simulink model "s_tanks_2_edit"  (R2021a)
settings: Solver=ode4  StartTime=0.0  StopTime=60  FixedStep=0.002  RelTol=1e-3  EnableMultiTasking=on
undefined symbols (not defined in the file or in its folder): Ao1, Ao2, At1, At2, g, Kff_2, Ki_1, Ki_2, Kp, Kp_1, Kp_2, L20, LR_1_MAX, MAX_L1_WDUP, MAX_L2_WDUP, TS, VMAX_AMP
settings Model: ExtModeTrigDuration=60000  Creator=MLevis  LastModifiedBy=tronc
settings SolverCC: AlgebraicLoopSolver=TrustRegion  PositivePriorityOrder=on
settings DataIOCC: LimitDataPoints=on  SaveFormat=Array  SignalLoggingSaveFormat=ModelDataLogs  ReturnWorkspaceOutputs=off
settings OptimizationCC: ExpressionDepthLimit=2147483647  InitFltsAndDblsToZero=on  LifeSpan=inf
settings DebuggingCC: SaveWithParameterizedLinksMsg=none  UnderspecifiedInitializationDetection=Classic  MergeDetectMultiDrivingBlocksExec=none  SolverPrmCheckMsg=warning  FcnCallInpInsideContextMsg=warning  StateNameClashWarn=warning  SFUnexpectedBacktrackingDiag=warning  SFNoUnconditionalDefaultTransitionDiag=warning  SFExecutionAtInitializationDiag=none  SFMachineParentedDataDiag=warning  ArithmeticOperatorsInVariantConditions=warning
settings HardwareCC: ProdBitPerPointer=32  ProdBitPerSizeT=32  ProdBitPerPtrDiffT=32  ProdLargestAtomicFloat=None  ProdIntDivRoundTo=Undefined  ProdEndianess=Unspecified  ProdWordSize=32  ProdHWDeviceType=32-bit Generic
settings ModelReferenceCC: PropagateSignalLabelsOutOfModel=off
settings SFSimCC: SimUseLocalCustomCode=off  CustomCodeUndefinedFunction=UseInterfaceOnly
settings RTWCC: Description=QuaRC Win32 Target  SystemTargetFile=quarc_windows.tlc  TemplateMakefile=quarc_default_tmf  RTWUseLocalCustomCode=off
settings CodeAppCC: StateflowObjectComments=on
settings STFCustomTargetCC: TargetFcnLib=ansi_tfl_tmw.mat  TargetPreCompLibLocation=C:\PROGRA~3\QUARC\lib\2012b\windows\release  CPPClassGenCompliant=on  UseToolchainInfoCompliant=off  SystemTargetFile=quarc_windows.tlc
settings GRTTargetCC: TargetFcnLib=ansi_tfl_tmw.mat  TargetPreCompLibLocation=C:\PROGRA~3\QUARC\lib\2012b\windows\release  TargetLangStandard=C89/C90 (ANSI)  ParMdlRefBuildCompliant=off  CompOptLevelCompliant=off  ConcurrentExecutionCompliant=off  CombineOutputUpdateFcns=off  MatFileLogging=off  GRTInterface=on  UseToolchainInfoCompliant=off  ExtMode=on  ExtModeMexFile=quarc_comm
settings ConfigComp: CovMetricSettings=dw  CovSaveCumulativeToWorkspaceVar=on  CovSaveSingleToWorkspaceVar=on  CovExternalEMLEnable=off

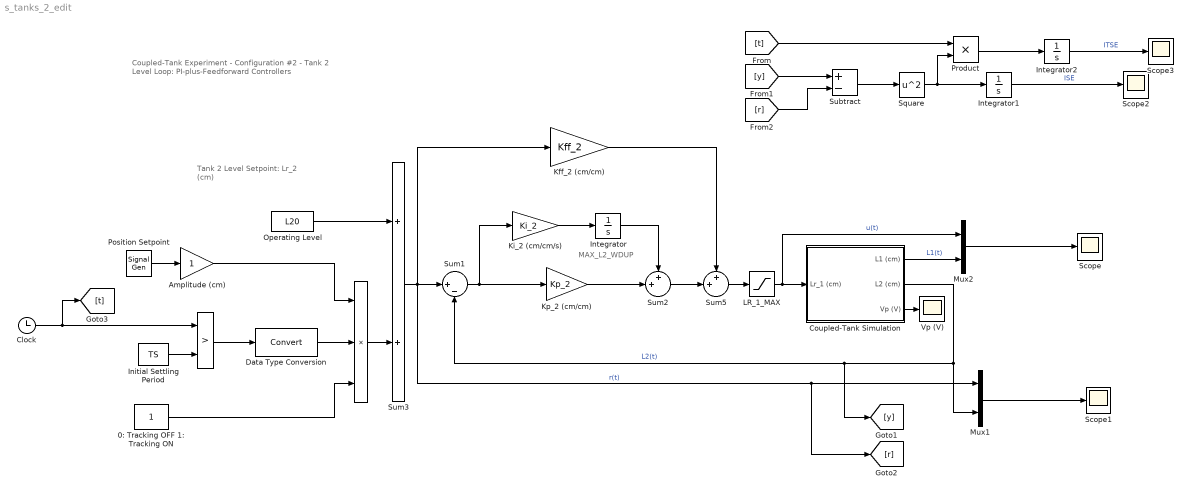
== system s_tanks_2_edit ==
  note: Coupled-Tank Experiment
      | - Configuration #2 -
      | Tank 2 Level Loop:
      | PI-plus-Feedforward Controllers
  note: Tank 2 Level Setpoint:
      | Lr_2 (cm)
  note: MAX_L2_WDUP
  "   " : Product  Inputs=3  InputSameDT=on  RndMeth=Zero  SaturateOnIntegerOverflow=on  OutDataTypeStr=Inherit: Same as first input
  "    " : RelationalOperator  Operator=>  RndMeth=Nearest  InputSameDT=on
  0: Tracking OFF 1: Tracking ON : Constant
  Amplitude (cm) : Gain  SaturateOnIntegerOverflow=on  OutDataTypeStr=Inherit: Same as input  ParamDataTypeStr=Inherit: Same as input
  Clock : Clock
  Coupled-Tank Simulation : Subsystem
  Data Type Conversion : DataTypeConversion
  Initial Settling Period : Constant  Value=TS
  Integrator : Integrator  LimitOutput=on  UpperSaturationLimit=MAX_L2_WDUP  LowerSaturationLimit=- MAX_L2_WDUP
  Integrator1 : Integrator
  Integrator2 : Integrator
  Kff_2 (cm/cm) : Gain  Gain=Kff_2  SaturateOnIntegerOverflow=on  OutDataTypeStr=Inherit: Same as input  ParamDataTypeStr=Inherit: Same as input
  Ki_2 (cm/cm/s) : Gain  Gain=Ki_2  SaturateOnIntegerOverflow=on  OutDataTypeStr=Inherit: Same as input  ParamDataTypeStr=Inherit: Same as input
  Kp_2 (cm/cm) : Gain  Gain=Kp_2  SaturateOnIntegerOverflow=on  OutDataTypeStr=Inherit: Same as input  ParamDataTypeStr=Inherit: Same as input
  LR_1_MAX : Saturate  UpperLimit=LR_1_MAX  LowerLimit=0
  Mux1 : Mux  Inputs=2
  Mux2 : Mux  Inputs=2
  Operating Level : Constant  Value=L20
  Position Setpoint : SignalGenerator  WaveForm=square  Frequency=0.018
  Product : Product
  Scope{,1..3} (4 alike) : Scope
  Square : Math  Operator=square  SaturateOnIntegerOverflow=on
  Subtract : Sum  Inputs=+-
  Sum1 : Sum  Inputs=|+-  InputSameDT=on  SaturateOnIntegerOverflow=on  OutDataTypeStr=Inherit: Same as first input
  Sum2 : Sum  Inputs=++|  InputSameDT=on  SaturateOnIntegerOverflow=on  OutDataTypeStr=Inherit: Same as first input
  Sum3 : Sum  InputSameDT=on  SaturateOnIntegerOverflow=on  OutDataTypeStr=Inherit: Same as first input
  Sum5 : Sum  Inputs=++|  InputSameDT=on  SaturateOnIntegerOverflow=on  OutDataTypeStr=Inherit: Same as first input
  Vp (V) : Scope
  wires:
  Mux2/1 -> Scope/1
  Position Setpoint/1 -> Amplitude (cm)/1
  0: Tracking OFF 1: Tracking ON/1 -> "   "/3
  "   "/1 -> Sum3/2
  Operating Level/1 -> Sum3/1
  Sum1/1 -> Kp_2 (cm/cm)/1, Ki_2 (cm/cm/s)/1
  Ki_2 (cm/cm/s)/1 -> Integrator/1
  Kp_2 (cm/cm)/1 -> Sum2/2
  Integrator/1 -> Sum2/1
  Sum2/1 -> Sum5/2
  Sum5/1 -> LR_1_MAX/1
  Kff_2 (cm/cm)/1 -> Sum5/1
  LR_1_MAX/1 -> Mux2/1, Coupled-Tank Simulation/1(Lr_1 (cm))  "u(t)"
  Mux1/1 -> Scope1/1
  Coupled-Tank Simulation/1(L1 (cm)) -> Mux2/2  "L1(t)"
  Initial Settling Period/1 -> "    "/2
  Clock/1 -> [t], "    "/1
  Amplitude (cm)/1 -> "   "/1
  "    "/1 -> Data Type Conversion/1
  Data Type Conversion/1 -> "   "/2
  Coupled-Tank Simulation/3(Vp (V)) -> Vp (V)/1
  [t] -> Product/1
  Integrator2/1 -> Scope3/1  "ITSE"
  Subtract/1 -> Square/1
  [r] -> Subtract/2
  [y] -> Subtract/1
  Product/1 -> Integrator2/1
  Square/1 -> Product/2, Integrator1/1
  Integrator1/1 -> Scope2/1  "ISE"
  Sum3/1 -> Kff_2 (cm/cm)/1, Sum1/1, [r], Mux1/1  "r(t)"
  Coupled-Tank Simulation/2(L2 (cm)) -> [y], Sum1/2, Mux1/2  "L2(t)"

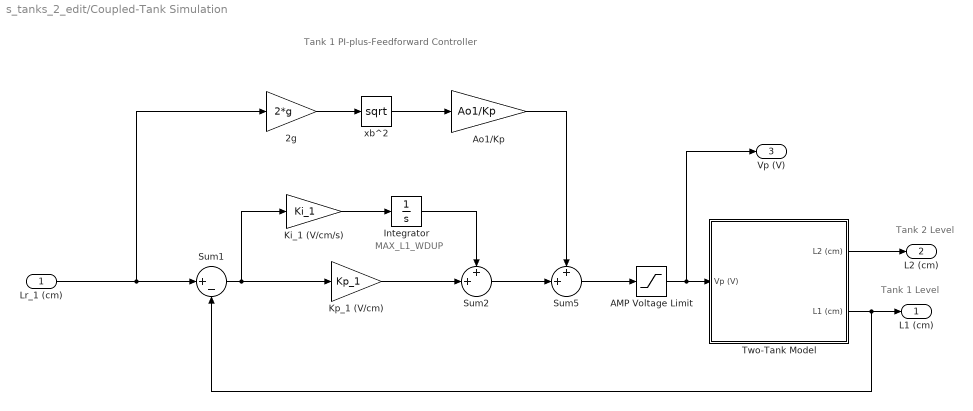
== system s_tanks_2_edit/Coupled-Tank Simulation ==
  note: Tank 1
      | PI-plus-Feedforward Controller
  note: Tank 1 Level
  note: Tank 2 Level
  note: MAX_L1_WDUP
  Lr_1 (cm) : Inport
  2g : Gain  Gain=2*g  SaturateOnIntegerOverflow=on  OutDataTypeStr=Inherit: Same as input  ParamDataTypeStr=Inherit: Same as input
  AMP Voltage Limit : Saturate  UpperLimit=VMAX_AMP  LowerLimit=0
  Ao1/Kp : Gain  Gain=Ao1/Kp  SaturateOnIntegerOverflow=on  OutDataTypeStr=Inherit: Same as input  ParamDataTypeStr=Inherit: Same as input
  Integrator : Integrator  LimitOutput=on  UpperSaturationLimit=MAX_L1_WDUP  LowerSaturationLimit=- MAX_L1_WDUP
  Ki_1 (V/cm/s) : Gain  Gain=Ki_1  SaturateOnIntegerOverflow=on  OutDataTypeStr=Inherit: Same as input  ParamDataTypeStr=Inherit: Same as input
  Kp_1 (V/cm) : Gain  Gain=Kp_1  SaturateOnIntegerOverflow=on  OutDataTypeStr=Inherit: Same as input  ParamDataTypeStr=Inherit: Same as input
  Sum1 : Sum  Inputs=|+-  InputSameDT=on  SaturateOnIntegerOverflow=on  OutDataTypeStr=Inherit: Same as first input
  Sum2 : Sum  Inputs=++|  InputSameDT=on  SaturateOnIntegerOverflow=on  OutDataTypeStr=Inherit: Same as first input
  Sum5 : Sum  Inputs=++|  InputSameDT=on  SaturateOnIntegerOverflow=on  OutDataTypeStr=Inherit: Same as first input
  Two-Tank Model : Subsystem
  xb^2 : Math  Operator=sqrt  SignedPower=on  SaturateOnIntegerOverflow=on
  L1 (cm) : Outport  InitialOutput=0
  L2 (cm) : Outport  Port=2  InitialOutput=0
  Vp (V) : Outport  Port=3  InitialOutput=0
  wires:
  Two-Tank Model/1(L2 (cm)) -> L2 (cm)/1
  Two-Tank Model/2(L1 (cm)) -> L1 (cm)/1, Sum1/2
  Ao1/Kp/1 -> Sum5/1
  xb^2/1 -> Ao1/Kp/1
  2g/1 -> xb^2/1
  Sum5/1 -> AMP Voltage Limit/1
  Sum2/1 -> Sum5/2
  AMP Voltage Limit/1 -> Two-Tank Model/1(Vp (V)), Vp (V)/1
  Integrator/1 -> Sum2/1
  Kp_1 (V/cm)/1 -> Sum2/2
  Ki_1 (V/cm/s)/1 -> Integrator/1
  Sum1/1 -> Kp_1 (V/cm)/1, Ki_1 (V/cm/s)/1
  Lr_1 (cm)/1 -> Sum1/1, 2g/1

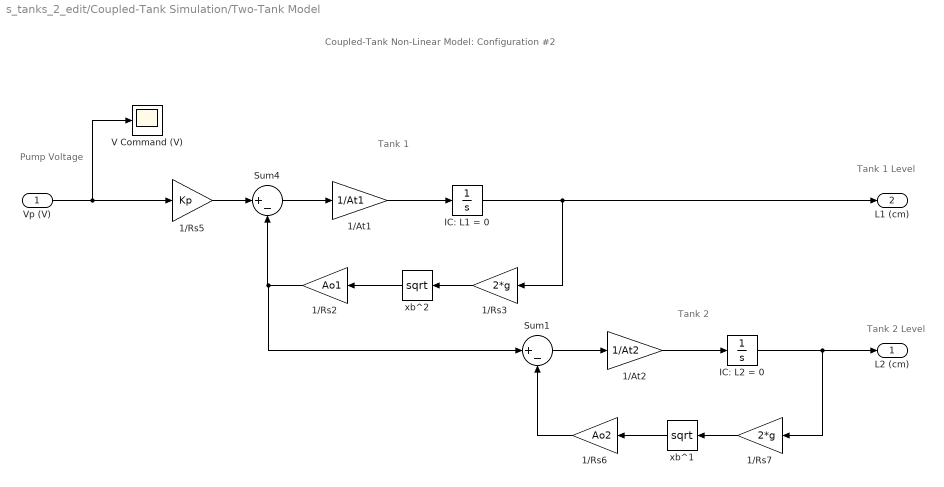
== system s_tanks_2_edit/Coupled-Tank Simulation/Two-Tank Model ==
  note: Pump
      | Voltage
  note: Tank 1 Level
  note: Tank 2 Level
  note: Tank 2
  note: Tank 1
  note: Coupled-Tank Non-Linear Model:
      | Configuration #2
  Vp (V) : Inport
  1/At1 : Gain  Gain=1/At1  SaturateOnIntegerOverflow=on  OutDataTypeStr=Inherit: Same as input  ParamDataTypeStr=Inherit: Same as input
  1/At2 : Gain  Gain=1/At2  SaturateOnIntegerOverflow=on  OutDataTypeStr=Inherit: Same as input  ParamDataTypeStr=Inherit: Same as input
  1/Rs2 : Gain  Gain=Ao1  SaturateOnIntegerOverflow=on  OutDataTypeStr=Inherit: Same as input  ParamDataTypeStr=Inherit: Same as input
  1/Rs3 : Gain  Gain=2*g  SaturateOnIntegerOverflow=on  OutDataTypeStr=Inherit: Same as input  ParamDataTypeStr=Inherit: Same as input
  1/Rs5 : Gain  Gain=Kp  SaturateOnIntegerOverflow=on  OutDataTypeStr=Inherit: Same as input  ParamDataTypeStr=Inherit: Same as input
  1/Rs6 : Gain  Gain=Ao2  SaturateOnIntegerOverflow=on  OutDataTypeStr=Inherit: Same as input  ParamDataTypeStr=Inherit: Same as input
  1/Rs7 : Gain  Gain=2*g  SaturateOnIntegerOverflow=on  OutDataTypeStr=Inherit: Same as input  ParamDataTypeStr=Inherit: Same as input
  IC: L1 = 0 : Integrator
  IC: L2 = 0 : Integrator
  Sum1 : Sum  Inputs=|+-  InputSameDT=on  SaturateOnIntegerOverflow=on  OutDataTypeStr=Inherit: Same as first input
  Sum4 : Sum  Inputs=|+-  InputSameDT=on  SaturateOnIntegerOverflow=on  OutDataTypeStr=Inherit: Same as first input
  V Command (V) : Scope
  xb^1 : Math  Operator=sqrt  SignedPower=on  SaturateOnIntegerOverflow=on
  xb^2 : Math  Operator=sqrt  SignedPower=on  SaturateOnIntegerOverflow=on
  L2 (cm) : Outport  InitialOutput=0
  L1 (cm) : Outport  Port=2  InitialOutput=0
  wires:
  1/Rs7/1 -> xb^1/1
  xb^1/1 -> 1/Rs6/1
  IC: L2 = 0/1 -> L2 (cm)/1, 1/Rs7/1
  1/At2/1 -> IC: L2 = 0/1
  Sum1/1 -> 1/At2/1
  1/Rs3/1 -> xb^2/1
  xb^2/1 -> 1/Rs2/1
  1/Rs2/1 -> Sum1/1, Sum4/2
  IC: L1 = 0/1 -> L1 (cm)/1, 1/Rs3/1
  1/At1/1 -> IC: L1 = 0/1
  Sum4/1 -> 1/At1/1
  1/Rs5/1 -> Sum4/1
  Vp (V)/1 -> 1/Rs5/1, V Command (V)/1
  1/Rs6/1 -> Sum1/2
